simulink model "CompliantModelSim"  (R2024b)
settings: Solver=VariableStepAuto  StartTime=0.0  StopTime=28.8659  MaxStep=.01  RelTol=1e-3
values from neighbouring files (symbols this model uses):
  B = 1/0.098736441    (= 10.1279729133)    [CompliantModel.m]
  B1 = 1.5*0.0007014    (= 0.0010521)    [CompliantModel.m]
  B2 = B1    (= 0.0010521)    [CompliantModel.m]
  Fc = 1.0*10.95    (= 10.95)    [CompliantModel.m]
  J1 = J    (= 2.7685e-06)    [CompliantModel.m]
  J2 = J    (= 2.7685e-06)    [CompliantModel.m]
  k1 = a*En/l1    (= 823.241162058)    [CompliantModel.m]
  k2 = a*En/l2    (= 823.241162058)    [CompliantModel.m]
  k3 = a*En/l3    (= 411.620581029)    [CompliantModel.m]
  Ke = Kt    (= 0.089999478)    [CompliantModel.m]
  Kt = 0.089999478    [CompliantModel.m]
  M = .17982    (= 0.17982)    [CompliantModel.m]
  R = 1.8    [CompliantModel.m]
  r = 0.011777    [CompliantModel.m]
  Tauc_1 = 1*10.95*TNm/100    (= 0.015851418414)    [CompliantModel.m]
  Tauc_2 = Tauc_1    (= 0.015851418414)    [CompliantModel.m]
settings Model: Creator=hjhje  LastModifiedBy=hjhje

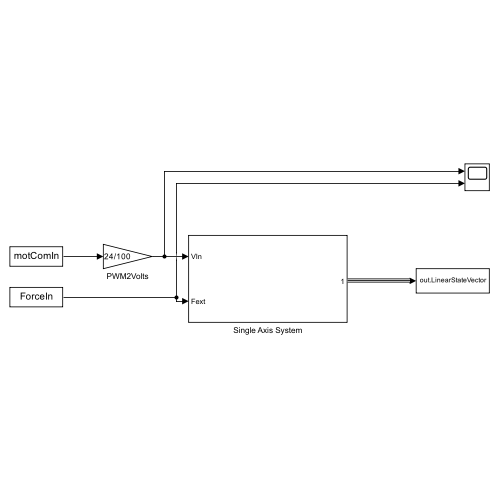
[thumbnail: Simulink's stored preview of the top-level diagram]
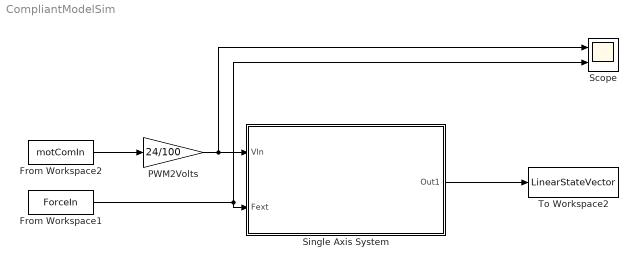
== system CompliantModelSim ==
  From Workspace1 : FromWorkspace  VariableName=ForceIn  SampleTime=-1  Interpolate=off  OutputAfterFinalValue=Holding final value
  From Workspace2 : FromWorkspace  VariableName=motComIn  SampleTime=-1  Interpolate=off  OutputAfterFinalValue=Holding final value
  PWM2Volts : Gain  Gain=24/100
  Scope : Scope  NumInputPorts=2
  Single Axis System : Subsystem
  To Workspace2 : ToWorkspace  VariableName=LinearStateVector  SaveFormat=Timeseries  SampleTime=-1
  wires:
  Single Axis System/1(Out1) -> To Workspace2/1
  From Workspace2/1 -> PWM2Volts/1
  From Workspace1/1 -> Scope/2, Single Axis System/2(Fext)
  PWM2Volts/1 -> Scope/1, Single Axis System/1(VIn)

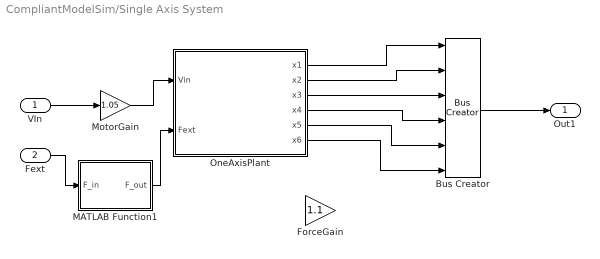
== system CompliantModelSim/Single Axis System ==
  VIn : Inport
  Fext : Inport  Port=2
  Bus Creator : BusCreator  Inputs=6
  ForceGain : Gain  Gain=1.1
  MATLAB Function1 : MATLAB Function  TreatAsAtomicUnit=on
  MotorGain : Gain  Gain=1.05
  OneAxisPlant : Subsystem
  Out1 : Outport
  wires:
  OneAxisPlant/1(x1) -> Bus Creator/1
  MotorGain/1 -> OneAxisPlant/1(Vin)
  OneAxisPlant/5(x5) -> Bus Creator/5
  OneAxisPlant/6(x6) -> Bus Creator/6
  OneAxisPlant/2(x2) -> Bus Creator/2
  OneAxisPlant/3(x3) -> Bus Creator/3
  OneAxisPlant/4(x4) -> Bus Creator/4
  Bus Creator/1 -> Out1/1
  VIn/1 -> MotorGain/1
  Fext/1 -> MATLAB Function1/1(F_in)
  MATLAB Function1/1(F_out) -> OneAxisPlant/2(Fext)

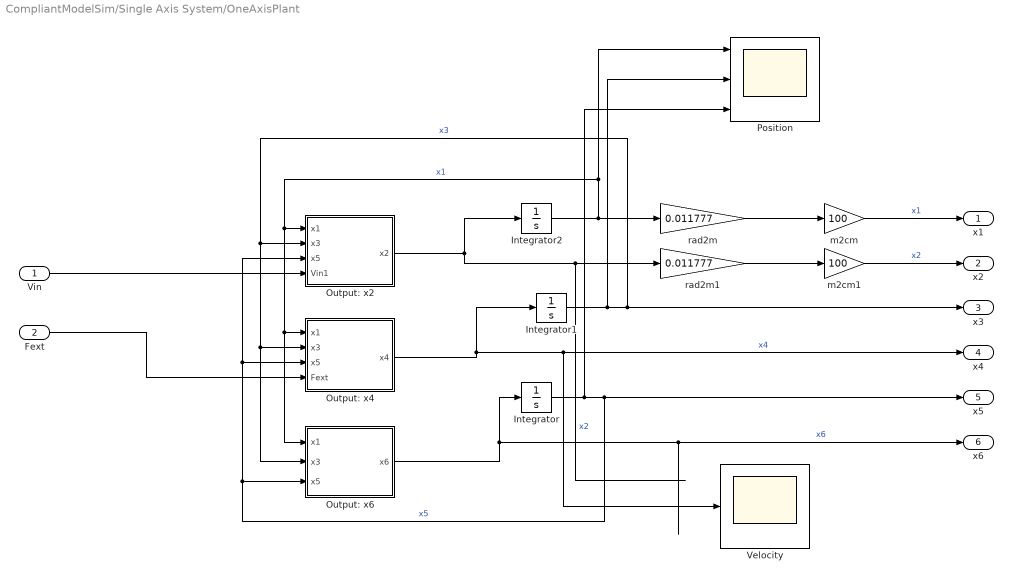
== system CompliantModelSim/Single Axis System/OneAxisPlant ==
  Vin : Inport
  Fext : Inport  Port=2
  Integrator : Integrator
  Integrator1 : Integrator
  Integrator2 : Integrator
  Output: x2 : Subsystem
  Output: x4 : Subsystem
  Output: x6 : Subsystem
  Position : Scope  NumInputPorts=3
  Velocity : Scope  NumInputPorts=3
  m2cm : Gain  Gain=100
  m2cm1 : Gain  Gain=100
  rad2m : Gain  Gain=0.011777
  rad2m1 : Gain  Gain=0.011777
  x1 : Outport
  x2 : Outport  Port=2
  x3 : Outport  Port=3
  x4 : Outport  Port=4
  x5 : Outport  Port=5
  x6 : Outport  Port=6
  wires:
  Output: x2/1(x2) -> rad2m1/1, Integrator2/1  "x2"
  Output: x4/1(x4) -> Integrator1/1, Velocity/2, x4/1  "x4"
  Output: x6/1(x6) -> Integrator/1, x6/1  "x6"
  Vin/1 -> Output: x2/4(Vin1)
  Integrator2/1 -> Position/1, Output: x6/1(x1), Output: x4/1(x1), Output: x2/1(x1), rad2m/1  "x1"
  Integrator1/1 -> Position/2, Output: x6/2(x3), Output: x4/2(x3), Output: x2/2(x3), x3/1  "x3"
  Integrator/1 -> Position/3, Output: x2/3(x5), Output: x4/3(x5), Output: x6/3(x5), x5/1  "x5"
  Fext/1 -> Output: x4/4(Fext)
  rad2m/1 -> m2cm/1
  rad2m1/1 -> m2cm1/1
  m2cm/1 -> x1/1  "x1"
  m2cm1/1 -> x2/1  "x2"

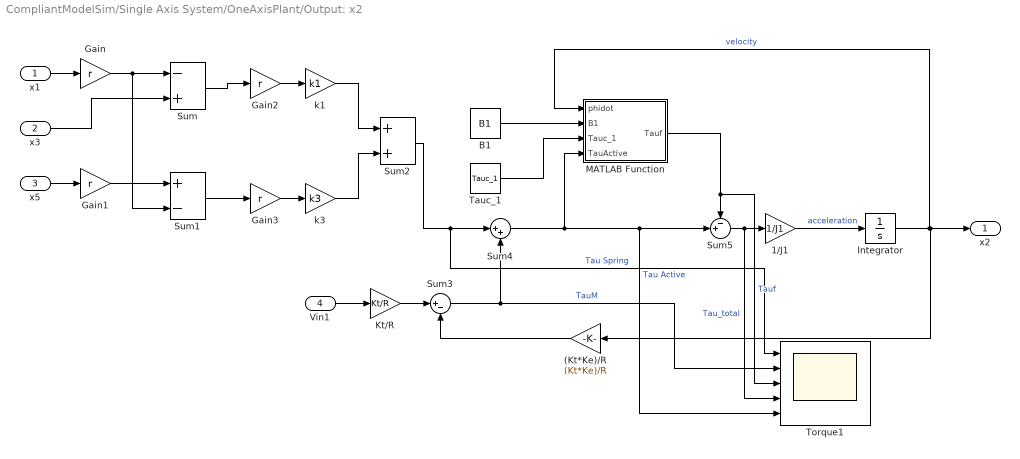
== system CompliantModelSim/Single Axis System/OneAxisPlant/Output: x2 ==
  x1 : Inport
  x3 : Inport  Port=2
  x5 : Inport  Port=3
  Vin1 : Inport  Port=4
  (Kt*Ke)/R : Gain  Gain=(Kt*Ke)/R
  1/J1 : Gain  Gain=1/J1
  B1 : Constant  Value=B1
  Gain{,1..3} (4 alike) : Gain  Gain=r
  Integrator : Integrator
  Kt/R : Gain  Gain=Kt/R
  MATLAB Function : MATLAB Function  TreatAsAtomicUnit=on
  Sum : Sum  Inputs=-+
  Sum1 : Sum  Inputs=+-
  Sum2 : Sum
  Sum3 : Sum  Inputs=|+-
  Sum4 : Sum  Inputs=|++
  Sum5 : Sum  Inputs=-+|
  Tauc_1 : Constant  Value=Tauc_1
  Torque1 : Scope  NumInputPorts=5
  k1 : Gain  Gain=k1
  k3 : Gain  Gain=k3
  x2 : Outport
  wires:
  x5/1 -> Gain1/1
  x1/1 -> Gain/1
  Gain/1 -> Sum1/2, Sum/1
  Gain1/1 -> Sum1/1
  x3/1 -> Sum/2
  Sum/1 -> Gain2/1
  Sum1/1 -> Gain3/1
  Gain2/1 -> k1/1
  Gain3/1 -> k3/1
  k1/1 -> Sum2/1
  k3/1 -> Sum2/2
  Vin1/1 -> Kt/R/1
  Sum2/1 -> Torque1/1, Sum4/1  "Tau Spring"
  Sum3/1 -> Sum4/2, Torque1/2  "TauM"
  Kt/R/1 -> Sum3/1
  B1/1 -> MATLAB Function/2(B1)
  Tauc_1/1 -> MATLAB Function/3(Tauc_1)
  Sum4/1 -> Torque1/5, Sum5/2, MATLAB Function/4(TauActive)  "Tau Active"
  MATLAB Function/1(Tauf) -> Torque1/3, Sum5/1  "Tauf"
  Sum5/1 -> Torque1/4, 1/J1/1  "Tau_total"
  Integrator/1 -> MATLAB Function/1(phidot), (Kt*Ke)/R/1, x2/1  "velocity"
  1/J1/1 -> Integrator/1  "acceleration"
  (Kt*Ke)/R/1 -> Sum3/2

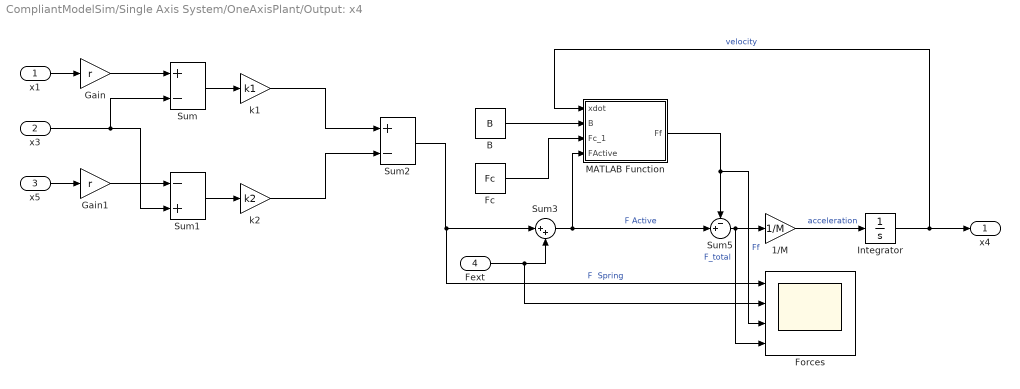
== system CompliantModelSim/Single Axis System/OneAxisPlant/Output: x4 ==
  x1 : Inport
  x3 : Inport  Port=2
  x5 : Inport  Port=3
  Fext : Inport  Port=4
  1/M : Gain  Gain=1/M
  B : Constant  Value=B
  Fc : Constant  Value=Fc
  Forces : Scope  NumInputPorts=4
  Gain : Gain  Gain=r
  Gain1 : Gain  Gain=r
  Integrator : Integrator
  MATLAB Function : MATLAB Function  TreatAsAtomicUnit=on
  Sum : Sum  Inputs=+-
  Sum1 : Sum  Inputs=-+
  Sum2 : Sum  Inputs=+-
  Sum3 : Sum  Inputs=|++
  Sum5 : Sum  Inputs=-+|
  k1 : Gain  Gain=k1
  k2 : Gain  Gain=k2
  x4 : Outport
  wires:
  x5/1 -> Gain1/1
  x1/1 -> Gain/1
  Sum2/1 -> Sum3/1, Forces/1  "F  Spring"
  MATLAB Function/1(Ff) -> Forces/3, Sum5/1  "Ff"
  Sum5/1 -> Forces/4, 1/M/1  "F_total"
  Integrator/1 -> MATLAB Function/1(xdot), x4/1  "velocity"
  1/M/1 -> Integrator/1  "acceleration"
  Gain/1 -> Sum/1
  x3/1 -> Sum1/2, Sum/2
  Sum/1 -> k1/1
  Gain1/1 -> Sum1/1
  Sum1/1 -> k2/1
  k2/1 -> Sum2/2
  k1/1 -> Sum2/1
  Fc/1 -> MATLAB Function/3(Fc_1)
  B/1 -> MATLAB Function/2(B)
  Fext/1 -> Forces/2, Sum3/2
  Sum3/1 -> MATLAB Function/4(FActive), Sum5/2  "F Active"

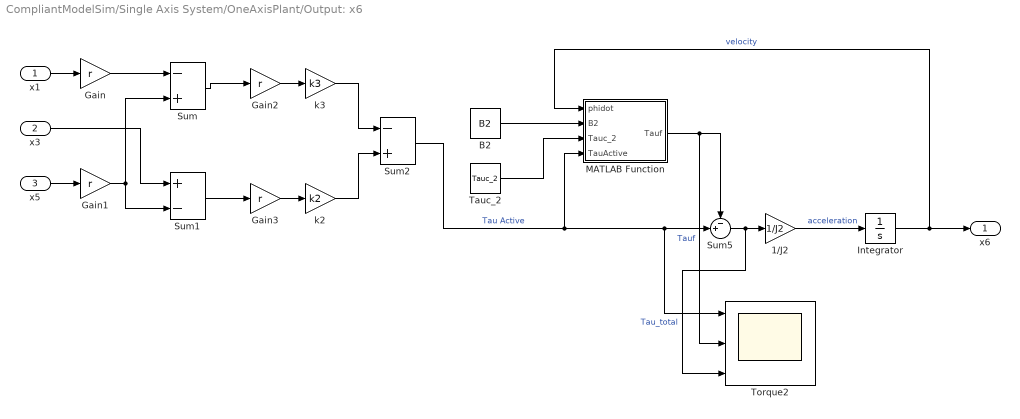
== system CompliantModelSim/Single Axis System/OneAxisPlant/Output: x6 ==
  x1 : Inport
  x3 : Inport  Port=2
  x5 : Inport  Port=3
  1/J2 : Gain  Gain=1/J2
  B2 : Constant  Value=B2
  Gain{,1..3} (4 alike) : Gain  Gain=r
  Integrator : Integrator
  MATLAB Function : MATLAB Function  TreatAsAtomicUnit=on
  Sum : Sum  Inputs=-+
  Sum1 : Sum  Inputs=+-
  Sum2 : Sum  Inputs=-+
  Sum5 : Sum  Inputs=-+|
  Tauc_2 : Constant  Value=Tauc_2
  Torque2 : Scope  NumInputPorts=3
  k2 : Gain  Gain=k2
  k3 : Gain  Gain=k3
  x6 : Outport
  wires:
  x5/1 -> Gain1/1
  x1/1 -> Gain/1
  Sum/1 -> Gain2/1
  Sum1/1 -> Gain3/1
  Gain2/1 -> k3/1
  Gain3/1 -> k2/1
  k3/1 -> Sum2/1
  k2/1 -> Sum2/2
  B2/1 -> MATLAB Function/2(B2)
  Tauc_2/1 -> MATLAB Function/3(Tauc_2)
  MATLAB Function/1(Tauf) -> Torque2/2, Sum5/1  "Tauf"
  Sum5/1 -> Torque2/3, 1/J2/1  "Tau_total"
  Integrator/1 -> MATLAB Function/1(phidot), x6/1  "velocity"
  1/J2/1 -> Integrator/1  "acceleration"
  x3/1 -> Sum1/1
  Gain1/1 -> Sum/2, Sum1/2
  Gain/1 -> Sum/1
  Sum2/1 -> Torque2/1, Sum5/2, MATLAB Function/4(TauActive)  "Tau Active"

== matlab function CompliantModelSim/Single Axis System/OneAxisPlant/Output: x4/MATLAB Function ==
  data: xdot input; Ff output; B input; Fc_1 input; FActive input
function Ff = fcn(xdot,B,Fc_1,FActive)
    Ff_tmp=B*xdot+sign(xdot)*Fc_1;
    if xdot>=-0.01 && xdot<=0.01 && abs(FActive)<=Fc_1
        Ff=FActive;
    else
        Ff=Ff_tmp;
    end
end

== matlab function CompliantModelSim/Single Axis System/OneAxisPlant/Output: x2/MATLAB Function ==
  data: phidot input; Tauf output; B1 input; Tauc_1 input; TauActive input
function Tauf = fcn(phidot,B1,Tauc_1,TauActive)
    Tauf_tmp=B1*phidot+sign(phidot)*Tauc_1;
    if phidot>=-0.01 && phidot<=0.01 && abs(TauActive)<=Tauc_1
        Tauf=TauActive;
    else
        Tauf=Tauf_tmp;
    end
end

== matlab function CompliantModelSim/Single Axis System/OneAxisPlant/Output: x6/MATLAB Function ==
  data: phidot input; Tauf output; B2 input; Tauc_2 input; TauActive input
function Tauf = fcn(phidot,B2,Tauc_2,TauActive)
    Tauf_tmp=B2*phidot+sign(phidot)*Tauc_2;
    if phidot>=-0.01 && phidot<=0.01 && abs(TauActive)<=Tauc_2
        Tauf=TauActive;
    else
        Tauf=Tauf_tmp;
    end
end

== matlab function CompliantModelSim/Single Axis System/MATLAB Function1 ==
  data: F_in input; F_out output
function F_out = fcn(F_in)

if (F_in > 0)
    scale = 1.;
else
    scale = 1;
end
% scale =.8;
F_out = scale*F_in;
